simulink model "dcmg"  (R2020a)
settings: Solver=VariableStepAuto  StartTime=0.0  StopTime=Inf  FixedStep=50e-6  RelTol=1e-3
PostLoadFcn:
  | , if any(exist('dsrtsu_mdlpostloadfcn', 'file') ~= 0), dsrtsu_mdlpostloadfcn('Execute', bdroot); end,
InitFcn:
  | , if any(exist('rtifpga_mdlclblib', 'file') ~= 0), rtifpga_mdlclblib('Init', bdroot); end,
model workspace (MAT data in the model file):
  FPGA_dcmg_1_Register_1_1_1_write : Simulink.Signal (value not decoded)
  FPGA_dcmg_1_Register_2_1_1_write : Simulink.Signal (value not decoded)
  FPGA_dcmg_1_Register_3_1_1_write : Simulink.Signal (value not decoded)
  FPGA_dcmg_1_Register_4_1_1_write : Simulink.Signal (value not decoded)
  FPGA_dcmg_1_Register_5_1_1_write : Simulink.Signal (value not decoded)
values from neighbouring files (symbols this model uses):
  den = [1, zeros(1,499)]    [params.m]
  fixedgain_i = 10*1000/(3*100)    (= 33.3333333333)    [param.m]    (also in params.m)
  fixedgain_ibat = 10*1000/(3*100)    (= 33.3333333333)    [params.m]
  fixedgain_ipv = 10*1000/(3*100)    (= 33.3333333333)    [params.m]
  fixedgain_v = 10*22000/(3*100*2.5)    (= 293.333333333)    [params.m]
  fixedgain_vdc = 10*22000/(3*100*2.5)    (= 293.333333333)    [param.m]    (also in params.m = 586.666666667)
  fixedgain_vpv = 10*10000/(3*100*2.5)    (= 133.333333333)    [params.m]
  gain_iavsi = 1    [params.m]
  gain_ibat = 1    [params.m]
  gain_ibvsi = 1    [params.m]
  gain_icvsi = 1    [params.m]
  gain_ioavsi = 1    [params.m]
  gain_iobvsi = 1    [params.m]
  gain_ipv = 1    [params.m]
  gain_sinwave = 0.3    [params.m]
  gain_vavsi = 1    [params.m]
  gain_vbvsi = 1    [params.m]
  gain_vcvsi = 1    [params.m]
  gain_vdc = 1    [param.m]    (also in params.m)
  gain_vpv = 1    [params.m]
  N = 10    [param.m]    (also in params.m = 100)
  num = 1/500*ones(1,500)    [params.m]
  offset_iavsi = 0.2    [params.m]
  offset_ibat = 0    [params.m]
  offset_ibvsi = 0.2    [params.m]
  offset_icvsi = 0.2    [params.m]
  offset_ioavsi = 0    [params.m]
  offset_iobvsi = 0    [params.m]
  offset_ipv = 0    [params.m]
  offset_vavsi = 0    [params.m]
  offset_vbvsi = 0    [params.m]
  offset_vcvsi = 0    [params.m]
  offset_vdc = 1.5    [param.m]    (also in params.m = 0)
  offset_vpv = 0    [params.m]
  v_dc_ref = 40    [param.m]    (also in params.m = 24)
libraries: xbsIndex_r4 x258, rti1202lib_adc_class1 x10, rtiproclib x9, simulink x5, rti1202lib_adc_class2 x2, rtifpgainterfacelib x1
(part 2 of 7)

== system dcmg/MPPT_system ==
  v_PV : Inport
  i_PV : Inport  Port=2
  v_DC : Inport  Port=3
  function : TriggerPort  TriggerType=function-call  VariantControl=Variant
  MATLAB Function : MATLAB Function  TreatAsAtomicUnit=on
  d : Outport
  wires:
  MATLAB Function/2(d) -> d/1
  i_PV/1 -> MATLAB Function/2(i)
  MATLAB Function/1(v_PandO) -> ?
  v_PV/1 -> MATLAB Function/1(v_pv)
  v_DC/1 -> MATLAB Function/3(v_dc)
  MATLAB Function/3(P) -> ?

== system dcmg/RTI Data ==
  RTI Data Store : Subsystem  Tag="struct('private',struct('version',struct('dsVer',uint32(2)),'access',struct('modified',['20-Dec-2024 14:14:36'],'type','Model','isPerm',1)),'public',struct('main',struct('data',[]),'sub',struct('name',{{'dcmg'}},'data',{{struct('TH',struct('thTaskInfo',struct('taskType',{'TIMER','HWINT','TMRINT','SWINT','GLINT'},'tasksNumOf',{1,3,0,0,0},'srcIds',{{'TIMERA'},{'FPGACL1FPGA_INTP0Ch1','FPGACL1FPGA_INTP0Ch0','FPGACL1FPGA_INTP0Ch2'},{},{},{}},'taskNames',{{['Timer Task 1']},{['PROC_INT_BL1 - interrupt_bat'],['PROC_INT_BL1 - interrupt_pv'],['PROC_INT_BL1 - interrupt_vsi']},{},{},{}})),'th_tc',struct('dataType',{'TASK','TASK','TASK','TASK'},'taskGroupId',{'','','',''},'taskGroupList',{{},{},{},{}},'taskSchedulingPolicy',{'FCFS','FCFS','FCFS','FCFS'},'taskType',{'TIMER','HWINT','HWINT','HWINT'},'blkh',{-1,['dcmg/PROC_INT_BL1 - interrupt_bat/Common Hardware' char(10) 'Interrupt Interface'],['dcmg/PROC_INT_BL1 - interrupt_pv/Common Hardware' char(10) 'Interrupt Interface'],['dcmg/PROC_INT_BL1 - interrupt_vsi/Common Hardware' char(10) 'Interrupt Interface']},'srcId',{'TIMERA','FPGACL1FPGA_INTP0Ch1','FPGACL1FPGA_INTP0Ch0','FPGACL1FPGA_INTP0Ch2'},'srcSgnName',{['Timer A interrupt'],['FPGA Type CL1 FPGA_INT Port 0 Channel 1'],['FPGA Type CL1 FPGA_INT Port 0 Channel 0'],['FPGA Type CL1 FPGA_INT Port 0 Channel 2']},'srcCpuName',{'','','',''},'taskName',{['Timer Task 1  [5e-05] s'],['PROC_INT_BL1 - interrupt_bat'],['PROC_INT_BL1 - interrupt_pv'],['PROC_INT_BL1 - interrupt_vsi']},'taskNameDisplayExt',{'','','',''},'smplTime',{5e-5,0,0,0},'smplTimeOffs',{0,0,0,0},'hasFixedPriority',{0,0,0,0},'priority',{4,1,2,3},'hasFixedOvc',{0,0,0,0},'ovcType',{1,1,1,1},'ovcMax',{1,1,1,1}),'tc_th',struct('dataType',{'TASK','TASK','TASK','TASK'},'taskGroupId',{'','','',''},'taskGroupList',{{},{},{},{}},'taskSchedulingPolicy',{'FCFS','FCFS','FCFS','FCFS'},'taskType',{'TIMER','HWINT','HWINT','HWINT'},'blkh',{-1,['dcmg/PROC_INT_BL1 - interrupt_bat/Common Hardware' char(10) 'Interrupt Interface'],['dcmg/PROC_INT_BL1 - interrupt_pv/Common Hardware' char(10) 'Interrupt Interface'],['dcmg/PROC_INT_BL1 - interrupt_vsi/Common Hardware' char(10) 'Interrupt Interface']},'srcId',{'TIMERA','FPGACL1FPGA_INTP0Ch1','FPGACL1FPGA_INTP0Ch0','FPGACL1FPGA_INTP0Ch2'},'srcSgnName',{['Timer A interrupt'],['FPGA Type CL1 FPGA_INT Port 0 Channel 1'],['FPGA Type CL1 FPGA_INT Port 0 Channel 0'],['FPGA Type CL1 FPGA_INT Port 0 Channel 2']},'srcCpuName',{'','','',''},'taskName',{['Timer Task 1  [5e-05] s'],['PROC_INT_BL1 - interrupt_bat'],['PROC_INT_BL1 - interrupt_pv'],['PROC_INT_BL1 - interrupt_vsi']},'taskNameDisplayExt',{'','','',''},'smplTime',{5e-5,0,0,0},'smplTimeOffs',{0,0,0,0},'hasFixedPriority',{0,0,0,0},'priority',{4,1,2,3},'hasFixedOvc',{0,0,0,0},'ovcType',{1,1,1,1},'ovcMax',{1,1,1,1}))}})))"  mask(RTI_DATA_STORE){}
      mask help:
      | RTI Data Store Block. This block is used by RTI to store internal model dependent data. Deleting this block will result in data loss.
      |
      | NEVER DELETE, COPY, OR MODIFY THIS BLOCK!
      mask Help:
      | RTI Data Store Block. This block is used by RTI to store internal model dependent data. Deleting this block will result in data loss.
      | 
      | NEVER DELETE, COPY, OR MODIFY THIS BLOCK!
      mask Display: text(0.5, 0.5, ' ', 'HorizontalAlignment', 'center');

== system dcmg/Subsystem ==
  v_dc : Inport
  i_bat : Inport  Port=2
  function : TriggerPort  TriggerType=function-call  VariantControl=Variant
  Discrete PID Controller : simulink/Continuous/PID Controller  Controller=PI  Form=Parallel  TimeDomain=Discrete-time  UseExternalTs=off  SampleTime=-1  IntegratorMethod=Forward Euler  FilterMethod=Forward Euler  ControllerParametersSource=internal  P=0.2  I=0.5  D=0  UseFilter=on  N=100  TunerSelectOption=Transfer Function Based (PID Tuner App)  InitialConditionSource=internal  InitialConditionForIntegrator=0  InitialConditionForFilter=0  DifferentiatorICPrevScaledInput=0  ExternalReset=none  TrackingMode=off  Kt=1  LimitOutput=on  UpperSaturationLimit=4  LowerSaturationLimit=-4  LinearizeAsGain=off  AntiWindupMode=none  Kb=1  POutMin=[]  POutMax=[]  IOutMin=[]  IOutMax=[]  DOutMin=[]  DOutMax=[]  NOutMin=[]  NOutMax=[]  SumOutMin=[]  SumOutMax=[]  SaturationOutMin=[]  SaturationOutMax=[]  PParamMin=[]  PParamMax=[]  IParamMin=[]  IParamMax=[]  DParamMin=[]  DParamMax=[]  NParamMin=[]  NParamMax=[]  KbParamMin=[]  KbParamMax=[]  KtParamMin=[]  KtParamMax=[]  KbOutMin=[]  KbOutMax=[]  KtOutMin=[]  KtOutMax=[]  IntegratorOutMin=[]  IntegratorOutMax=[]  FilterOutMin=[]  FilterOutMax=[]  SumI1OutMin=[]  SumI1OutMax=[]  SumI2OutMin=[]  SumI2OutMax=[]  SumI3OutMin=[]  SumI3OutMax=[]  SumI4OutMin=[]  SumI4OutMax=[]  SumDOutMin=[]  SumDOutMax=[]  DifferentiatorOutMin=[]  DifferentiatorOutMax=[]  FilterDiffOutCoefMin=[]  FilterDiffOutCoefMax=[]  ReciprocalOutMin=[]  ReciprocalOutMax=[]  SumDenOutMin=[]  SumDenOutMax=[]  SumNumOutMin=[]  SumNumOutMax=[]  DivideOutMin=[]  DivideOutMax=[]  UdiffTsProdOutMin=[]  UdiffTsProdOutMax=[]  NTsProdOutMin=[]  NTsProdOutMax=[]  UintegralTsProdOutMin=[]  UintegralTsProdOutMax=[]  UngainTsProdOutMin=[]  UngainTsProdOutMax=[]  IntegratorContinuousStateAttributes=''  IntegratorStateMustResolveToSignalObject=off  IntegratorRTWStateStorageClass=Auto  FilterContinuousStateAttributes=''  FilterStateMustResolveToSignalObject=off  FilterRTWStateStorageClass=Auto  ParallelPVariant=InternalParameters  IdealPVariant=Disabled  IVariant=InternalParameters  DVariant=Disabled  IntegratorVariant=Discrete  SatVariant=Enabled  AWVariant=Passthrough  PCopyVariant=Disabled  TRVariant=Disabled  FdbkBlocksVariant=Forward  IdealPFdbkVariant=Disabled  SatFdbkVariant=Disabled  DerivativeFilterVariant=Disabled  NVariant=Disabled  NCopyVariant=Disabled_SignalSpec  FilterICVariant=Disabled  IntegratorICVariant=InternalICs  ExternalResetVariant=Disabled  TRSumVariant=Passthrough  SumFdbkVariant=Disabled  SumVariant=Sum_PI  TsampFilterVariant=InternalTs  TsampNgainVariant=Passthrough  TsampIntegralVariant=Passthrough
  Discrete PID Controller1 : simulink/Continuous/PID Controller  Controller=PI  Form=Parallel  TimeDomain=Discrete-time  UseExternalTs=off  SampleTime=-1  IntegratorMethod=Forward Euler  FilterMethod=Forward Euler  ControllerParametersSource=internal  P=10  I=10  D=0  UseFilter=on  N=100  TunerSelectOption=Transfer Function Based (PID Tuner App)  InitialConditionSource=internal  InitialConditionForIntegrator=0  InitialConditionForFilter=0  DifferentiatorICPrevScaledInput=0  ExternalReset=none  TrackingMode=off  Kt=1  LimitOutput=on  UpperSaturationLimit=.99  LowerSaturationLimit=0.01  LinearizeAsGain=on  AntiWindupMode=none  Kb=1  POutMin=[]  POutMax=[]  IOutMin=[]  IOutMax=[]  DOutMin=[]  DOutMax=[]  NOutMin=[]  NOutMax=[]  SumOutMin=[]  SumOutMax=[]  SaturationOutMin=[]  SaturationOutMax=[]  PParamMin=[]  PParamMax=[]  IParamMin=[]  IParamMax=[]  DParamMin=[]  DParamMax=[]  NParamMin=[]  NParamMax=[]  KbParamMin=[]  KbParamMax=[]  KtParamMin=[]  KtParamMax=[]  KbOutMin=[]  KbOutMax=[]  KtOutMin=[]  KtOutMax=[]  IntegratorOutMin=[]  IntegratorOutMax=[]  FilterOutMin=[]  FilterOutMax=[]  SumI1OutMin=[]  SumI1OutMax=[]  SumI2OutMin=[]  SumI2OutMax=[]  SumI3OutMin=[]  SumI3OutMax=[]  SumI4OutMin=[]  SumI4OutMax=[]  SumDOutMin=[]  SumDOutMax=[]  DifferentiatorOutMin=[]  DifferentiatorOutMax=[]  FilterDiffOutCoefMin=[]  FilterDiffOutCoefMax=[]  ReciprocalOutMin=[]  ReciprocalOutMax=[]  SumDenOutMin=[]  SumDenOutMax=[]  SumNumOutMin=[]  SumNumOutMax=[]  DivideOutMin=[]  DivideOutMax=[]  UdiffTsProdOutMin=[]  UdiffTsProdOutMax=[]  NTsProdOutMin=[]  NTsProdOutMax=[]  UintegralTsProdOutMin=[]  UintegralTsProdOutMax=[]  UngainTsProdOutMin=[]  UngainTsProdOutMax=[]  IntegratorContinuousStateAttributes=''  IntegratorStateMustResolveToSignalObject=off  IntegratorRTWStateStorageClass=Auto  FilterContinuousStateAttributes=''  FilterStateMustResolveToSignalObject=off  FilterRTWStateStorageClass=Auto  ParallelPVariant=InternalParameters  IdealPVariant=Disabled  IVariant=InternalParameters  DVariant=Disabled  IntegratorVariant=Discrete  SatVariant=Enabled  AWVariant=Passthrough  PCopyVariant=Disabled  TRVariant=Disabled  FdbkBlocksVariant=Forward  IdealPFdbkVariant=Disabled  SatFdbkVariant=Disabled  DerivativeFilterVariant=Disabled  NVariant=Disabled  NCopyVariant=Disabled_SignalSpec  FilterICVariant=Disabled  IntegratorICVariant=InternalICs  ExternalResetVariant=Disabled  TRSumVariant=Passthrough  SumFdbkVariant=Disabled  SumVariant=Sum_PI  TsampFilterVariant=InternalTs  TsampNgainVariant=Passthrough  TsampIntegralVariant=Passthrough
  Sum : Sum  Inputs=|+-
  Sum1 : Sum  Inputs=|+-
  v_DC_ref : Constant  Value=v_dc_ref
  y1 : Outport
  wires:
  v_DC_ref/1 -> Sum/1
  Sum1/1 -> Discrete PID Controller1/1
  Sum/1 -> Discrete PID Controller/1
  Discrete PID Controller/1 -> Sum1/1
  v_dc/1 -> Sum/2
  Discrete PID Controller1/1 -> y1/1
  i_bat/1 -> Sum1/2

== system dcmg/Subsystem1 ==
  In1 : Inport
  function : TriggerPort  TriggerType=function-call  VariantControl=Variant
  Constant1 : Constant  Value=-2*pi/3
  Constant2 : Constant  Value=2*pi/3
  Constant3 : Constant
  Constant4 : Constant
  Constant5 : Constant
  Gain : Gain  Gain=gain_sinwave
  Gain1 : Gain  Gain=gain_sinwave
  Gain2 : Gain  Gain=gain_sinwave
  Sin : Trigonometry
  Sin1 : Trigonometry
  Sin2 : Trigonometry
  Sum{,1..4} (5 alike) : Sum  Inputs=|++
  Out1 : Outport
  Out2 : Outport  Port=2
  Out3 : Outport  Port=3
  wires:
  Sin/1 -> Sum2/1
  In1/1 -> Sin/1, Sum1/1, Sum/1
  Constant1/1 -> Sum/2
  Constant2/1 -> Sum1/2
  Sum/1 -> Sin1/1
  Sum1/1 -> Sin2/1
  Sin1/1 -> Sum3/1
  Sin2/1 -> Sum4/1
  Sum2/1 -> Gain/1
  Sum4/1 -> Gain2/1
  Gain/1 -> Out1/1
  Gain2/1 -> Out3/1
  Gain1/1 -> Out2/1
  Sum3/1 -> Gain1/1
  Constant3/1 -> Sum2/2
  Constant4/1 -> Sum3/2
  Constant5/1 -> Sum4/2
